simulink model "State_of_Charge"  (R2020a)
settings: Solver=VariableStepAuto  StartTime=0.0  StopTime=10.0  RelTol=1e-3
libraries: simulink x2
settings Model: Creator=akash  LastModifiedBy=akash

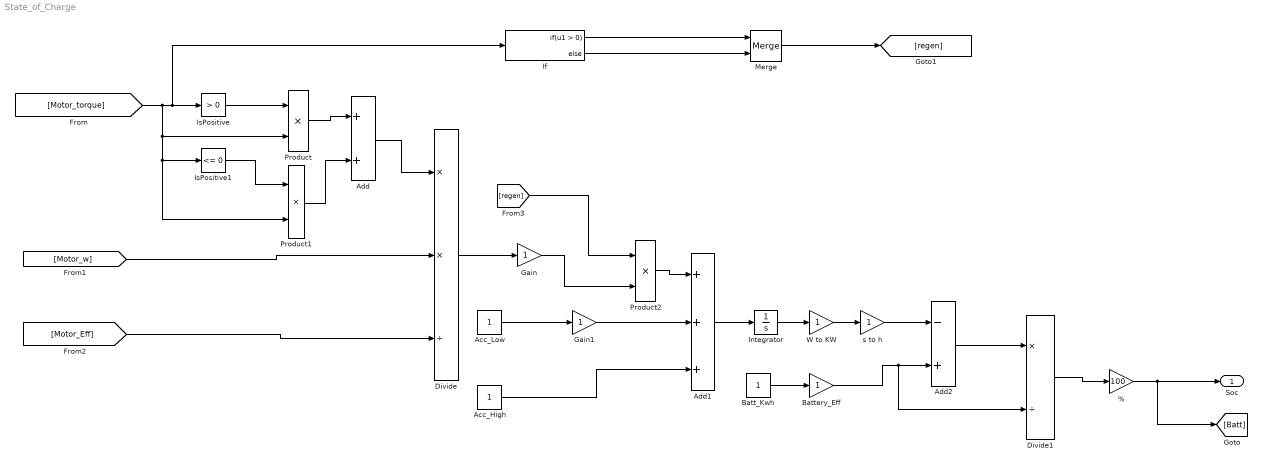
== system State_of_Charge ==
  % : Gain  Gain=100
  Acc_High : Constant
  Acc_Low : Constant
  Add : Sum
  Add1 : Sum  Inputs=+++
  Add2 : Sum  Inputs=-+
  Batt_Kwh : Constant
  Battery_Eff : Gain
  Divide : Product  Inputs=**/
  Divide1 : Product  Inputs=*/
  Gain : Gain
  Gain1 : Gain
  If : If
  Integrator : Integrator
  IsPositive : simulink/Logic and Bit Operations/Compare To Zero  relop=>  OutDataTypeStr=boolean
  IsPositive1 : simulink/Logic and Bit Operations/Compare To Zero  relop=<=  OutDataTypeStr=boolean
  Merge : Merge
  Product : Product
  Product1 : Product
  Product2 : Product
  W to KW : Gain
  s to h : Gain
  Soc : Outport
  wires:
  Product/1 -> Add/1
  Product1/1 -> Add/2
  IsPositive/1 -> Product/1
  IsPositive1/1 -> Product1/1
  Add/1 -> Divide/1
  [Motor_torque] -> Product1/2, IsPositive1/1, Product/2, If/1, IsPositive/1
  [Motor_w] -> Divide/2
  [Motor_Eff] -> Divide/3
  Divide/1 -> Gain/1
  [regen] -> Product2/1
  Gain/1 -> Product2/2
  Gain1/1 -> Add1/2
  Acc_Low/1 -> Gain1/1
  Acc_High/1 -> Add1/3
  W to KW/1 -> s to h/1
  s to h/1 -> Add2/1
  Add1/1 -> Integrator/1
  Integrator/1 -> W to KW/1
  Batt_Kwh/1 -> Battery_Eff/1
  Battery_Eff/1 -> Divide1/2, Add2/2
  Add2/1 -> Divide1/1
  Divide1/1 -> %/1
  %/1 -> [Batt], Soc/1
  If/1 -> Merge/1
  If/2 -> Merge/2
  Merge/1 -> [regen]
  Product2/1 -> Add1/1
